simulink model "CE1simulink"  (R2025b)
settings: Solver=VariableStepAuto  StartTime=0.0  StopTime=240.0  FixedStep=0.1  RelTol=1e-3
model workspace (MAT data in the model file):
  Ts = 0.1
settings Model: Creator=kristinanordang  LastModifiedBy=kristinanordang

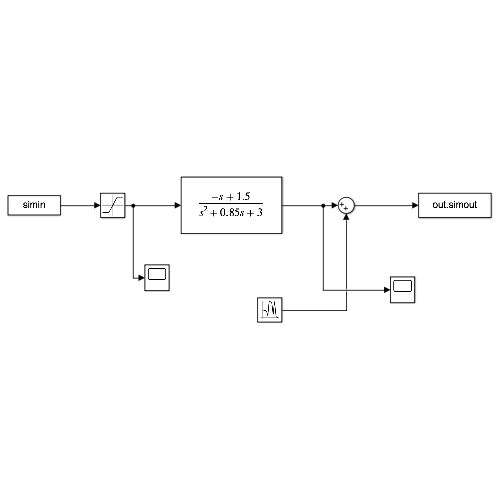
[thumbnail: Simulink's stored preview of the top-level diagram]
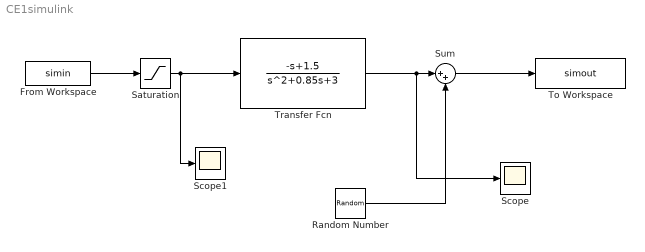
== system CE1simulink ==
  From Workspace : FromWorkspace  VariableName=simin  SampleTime=Ts
  Random Number : RandomNumber  Variance=0.01  SampleTime=Ts
  Saturation : Saturate  UpperLimit=0.9  LowerLimit=-0.9
  Scope : Scope
      settings: ActiveDisplayYMinimum=-1.0201189042624448  ActiveDisplayYMaximum=0.96924074666932425
  Scope1 : Scope
      settings: ActiveDisplayYMinimum=-0.2184191787587545  ActiveDisplayYMaximum=1.0263766419932703
  Sum : Sum  Inputs=|++
  To Workspace : ToWorkspace  VariableName=simout  SaveFormat=Timeseries  SampleTime=Ts
  Transfer Fcn : TransferFcn  Numerator=[-1 1.5]  Denominator=[1 0.85 3]
  wires:
  Transfer Fcn/1 -> Scope/1, Sum/1
  Random Number/1 -> Sum/2
  Saturation/1 -> Scope1/1, Transfer Fcn/1
  Sum/1 -> To Workspace/1
  From Workspace/1 -> Saturation/1
